simulink model "delayed_mpc_model"  (R2019a)
settings: Solver=FixedStepAuto  StartTime=0.0  StopTime=Tfinal  RelTol=1e-3
values from neighbouring files (symbols this model uses):
  A = [-0.0285 -0.0014; -0.0371 -0.1476]    [model.m]
  DCLINK_Cap = 1000e-12    (= 1e-09)    [mpc_model_parameters.m]    (also in mpc_model_parameters_dual_module.m = 0.001)
  FaultTime = 50    [mpc_model_parameters.m]
  FluxPM = MeanInducedVoltagePeak/(2*pi*100)    [mpc_model_parameters.m]    (also in mpc_model_parameters_dual_module.m)
  Inertia = 1e-2    (= 0.01)    [mpc_model_parameters.m]    (also in mpc_model_parameters_dual_module.m)
  iqrated = Trated/(1.5*PolePairs*FluxPM)    [mpc_model_parameters.m]    (also in mpc_model_parameters_dual_module.m)
  MeanLq = (1/12)*(Module1Phase_A_Lq+Module1Phase_B_Lq+Module1Phase_C_Lq+     Module2Phase_A_Lq+Module2Phase_B_Lq+Module2Phase_C_Lq+     Module3Phase_A_Lq+Module3Phase_B_Lq+Module3Phase_C_Lq+     Module4Phase_A_Lq+Module4Phase_B_Lq+Module4Phase_C_Lq)    [mpc_model_parameters.m]    (also in mpc_model_parameters_dual_module.m)
  PolePairs = 10    [mpc_model_parameters.m]    (also in mpc_model_parameters_dual_module.m)
  Rin = 1e-3    (= 0.001)    [mpc_model_parameters.m]    (also in mpc_model_parameters_dual_module.m)
  Rs = 0.531    [Loss_Distribution.m]    (also in MPC_id_iq.m; mpc_model_parameters.m = 0.321; mpc_model_parameters_dual_module.m = 0.539)
  Sampling_time = 1e-6    (= 1e-06)    [mpc_model_parameters.m]    (also in mpc_model_parameters_dual_module.m)
  SpeedRef1 = 50    [mpc_model_parameters.m]    (also in mpc_model_parameters_dual_module.m = 35)
  SpeedRef2 = 100    [mpc_model_parameters.m]    (also in mpc_model_parameters_dual_module.m = 35)
  SpeedRefUpdateTime = 0.25    [mpc_model_parameters.m]    (also in mpc_model_parameters_dual_module.m = 1.75)
  Tload1 = 5    [mpc_model_parameters.m]    (also in mpc_model_parameters_dual_module.m = 30)
  Tload2 = 10    [mpc_model_parameters.m]    (also in mpc_model_parameters_dual_module.m = 63.6619772368)
  TloadUpdateTime = 0.5    [mpc_model_parameters.m]    (also in mpc_model_parameters_dual_module.m)
  Vdc = 50    [mpc_model_parameters.m]    (also in mpc_model_parameters_dual_module.m = 40)
  Vin = Vdc + Rin*(Pout/Vdc)    (= 50.04)    [mpc_model_parameters.m]    (also in mpc_model_parameters_dual_module.m = 40.05)
  ViscousFriction = 1e-3    (= 0.001)    [mpc_model_parameters.m]    (also in mpc_model_parameters_dual_module.m)
undefined symbols (not defined in the file or in its folder): DiscIntNeverNeededParam
libraries: powerlib x16, dspswit3 x7, dspsigops x4, simulink x3, powerlib_meascontrol x2
settings Model: Creator=hakan  LastModifiedBy=hakan
settings SolverCC: ZeroCrossAlgorithm=Adaptive
settings DebuggingCC: IgnoredZcDiagnostic=none

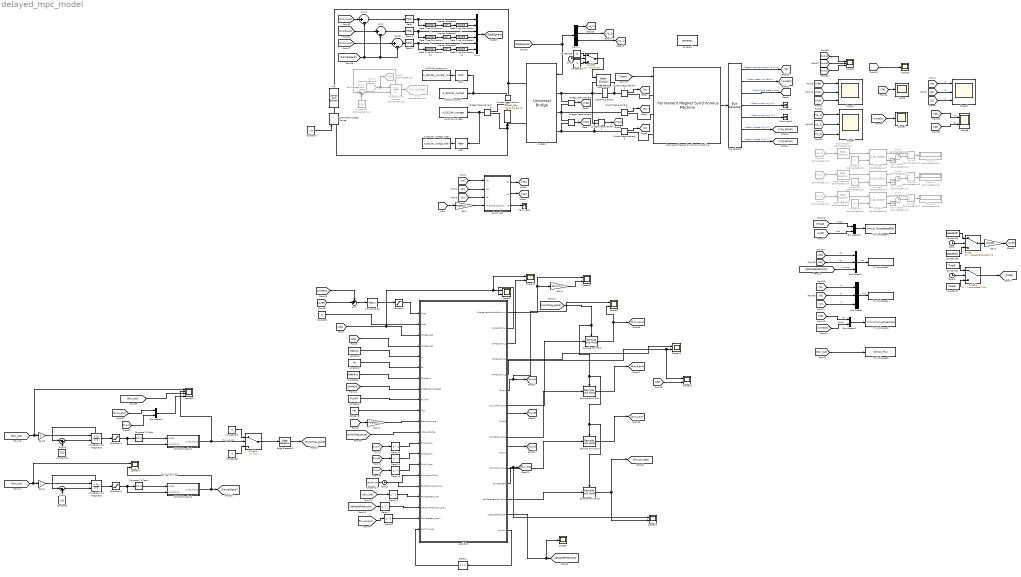
== system delayed_mpc_model ==
  A_DCLINK_current : ToWorkspace  VariableName=A_DCLINK_current  SaveFormat=Structure With Time  SampleTime=-1
  A_DCLINK_current_rms : ToWorkspace  VariableName=A_DCLINK_current_rms  SaveFormat=Structure With Time  SampleTime=-1
  A_DCLINK_voltage : ToWorkspace  VariableName=A_DCLINK_voltage  SaveFormat=Structure With Time  SampleTime=-1
  A_DCLINK_voltage_mean : ToWorkspace  VariableName=A_DCLINK_voltage_mean  SaveFormat=Structure With Time  SampleTime=-1
  Bus Creator : BusCreator  Inputs=3
  Bus Creator1 : BusCreator  Inputs=3
  Bus Creator2 : BusCreator  Inputs=2
  Bus Creator3 : BusCreator  Inputs=2
  Bus Creator4 : BusCreator  Inputs=2
  Bus Selector : BusSelector  OutputSignals=Electromagnetic torque Te (N*m),Rotor speed wm (rad/s),Rotor angle thetam (rad),Stator current is_q (A),Stator current is_d (A),Stator voltage Vs_q (V),Stator voltage Vs_d (V)
  Clock{,1..3} (4 alike) : Clock
  Clock4 : Clock  Commented=on
  Clock5 : Clock  Commented=on
  Clock6 : Clock  Commented=on
  Compare To Zero : simulink/Logic and Bit Operations/Compare To Zero  relop===  OutDataTypeStr=boolean
  Compare To Zero1 : simulink/Logic and Bit Operations/Compare To Zero  relop===  OutDataTypeStr=boolean
  Constant : Constant  Value=Vin
  Constant1 : Constant  Value=0
  Constant10 : Constant  Value=SpeedRef1
  Constant11 : Constant  Value=SpeedRef2
  Constant12 : Constant  Value=Tload2
  Constant15 : Constant  Value=0
  Constant16 : Constant
  Constant17 : Constant  Value=FaultTime
  Constant18 : Constant  Commented=on  Value=0
  Constant19 : Constant  Commented=on  Value=0
  Constant2 : Constant  Value=MeanLq
  Constant20 : Constant  Commented=on  Value=0
  Constant24 : Constant  Value=1.02
  Constant26 : Constant  Commented=on  Value=1.04
  Constant29 : Constant  Value=0
  Constant3 : Constant  Value=1.02
  Constant30 : Constant
  Constant5 : Constant  Value=Rs
  Constant6 : Constant  Value=PolePairs
  Constant7 : Constant  Value=FluxPM
  Constant8 : Constant  Value=Tload1
  Constant9 : Constant  Value=Vdc
  Controlled Voltage Source : powerlib/Electrical Sources/Controlled Voltage Source  Initialize=on  Source_Type=DC  Amplitude=Vin  Phase=0  Frequency=0  Measurements=None
      settings: SourceProductName=Simscape Electrical
  Counter : dspswit3/Counter  Commented=on  Direction=Up  CountEvent=Rising edge  CounterSize=User defined  MaxCount=9999999999999999999  InitialCount=0  Output=Count and Hit  HitValue=32  ResetInput=on  SamplesPerFrame=1  Ts=1  CntDtype=double  HitDtype=Logical
  Counter1 : dspswit3/Counter  Commented=on  Direction=Up  CountEvent=Rising edge  CounterSize=User defined  MaxCount=9999999999999999999  InitialCount=0  Output=Count and Hit  HitValue=32  ResetInput=on  SamplesPerFrame=1  Ts=1  CntDtype=double  HitDtype=Logical
  Counter2 : dspswit3/Counter  Commented=on  Direction=Up  CountEvent=Rising edge  CounterSize=User defined  MaxCount=9999999999999999999  InitialCount=0  Output=Count and Hit  HitValue=32  ResetInput=on  SamplesPerFrame=1  Ts=1  CntDtype=double  HitDtype=Logical
  Current Measurement{,1..3} (4 alike) : powerlib/Measurements/Current Measurement  PhasorSimulation=off  OutputType=Complex  PSBequivalent=0
      settings: SourceProductName=Simscape Electrical
  DCLINK_Cap : powerlib/Elements/Series RLC Branch  LConnTagsString=__new0  RConnTagsString=__new0  BranchType=C  Resistance=1  Inductance=1e-3  SetiL0=off  InitialCurrent=0  Capacitance=DCLINK_Cap  Setx0=on  InitialVoltage=Vin  Measurements=None
      settings: SourceProductName=Simscape Electrical
  Data Type Conversion10 : DataTypeConversion  OutDataTypeStr=boolean
  Data Type Conversion11 : DataTypeConversion  OutDataTypeStr=double
  Data Type Conversion6 : DataTypeConversion  OutDataTypeStr=boolean
  Data Type Conversion7 : DataTypeConversion  OutDataTypeStr=double
  Data Type Conversion8 : DataTypeConversion  OutDataTypeStr=boolean
  Data Type Conversion9 : DataTypeConversion  OutDataTypeStr=double
  Delay{1..2,5,11..14} (7 alike) : Delay  DelayLength=1
  Demux : Demux  Outputs=6
  Discrete-Time Integrator : DiscreteIntegrator  Commented=on  ExternalReset=falling  SampleTime=-1  ShowStatePort=on  ICPrevOutput=DiscIntNeverNeededParam  ICPrevScaledInput=DiscIntNeverNeededParam
  Discrete-Time Integrator1 : DiscreteIntegrator  ExternalReset=falling  SampleTime=Sampling_time  UpperSaturationLimit=1  LowerSaturationLimit=0  ShowStatePort=on  ICPrevOutput=DiscIntNeverNeededParam  ICPrevScaledInput=DiscIntNeverNeededParam
  Discrete-Time Integrator2 : DiscreteIntegrator  ExternalReset=falling  SampleTime=Sampling_time  UpperSaturationLimit=1  LowerSaturationLimit=0  ShowStatePort=on  ICPrevOutput=DiscIntNeverNeededParam  ICPrevScaledInput=DiscIntNeverNeededParam
  Display1 : Display  Commented=on
  Display2 : Display  Commented=on
  Display3 : Display  Commented=on
  Divide : Product  Commented=on  Inputs=*/
  Divide1 : Product  Commented=on  Inputs=*/
  Divide2 : Product  Commented=on  Inputs=*/
  Edge Detector : dspswit3/Edge Detector  Commented=on  InputProcessing=Columns as channels (frame based)
      settings: SourceProductName=DSP System Toolbox  SourceProductBaseCode=DS
  Edge Detector1 : dspswit3/Edge Detector  Commented=on  InputProcessing=Columns as channels (frame based)
      settings: SourceProductName=DSP System Toolbox  SourceProductBaseCode=DS
  Edge Detector2 : dspswit3/Edge Detector  Commented=on  InputProcessing=Columns as channels (frame based)
      settings: SourceProductName=DSP System Toolbox  SourceProductBaseCode=DS
  Edge Detector3 : dspswit3/Edge Detector  InputProcessing=Columns as channels (frame based)
      settings: SourceProductName=DSP System Toolbox  SourceProductBaseCode=DS
  From40 : From  Commented=on  GotoTag=va_1
  From41 : From  Commented=on  GotoTag=vb_1
  From42 : From  Commented=on  GotoTag=vc_1
  From72 : From  Commented=on  GotoTag=fsw_out
  Gain : Gain  Gain=PolePairs
  Gain1 : Gain  Gain=2*pi/60
  Gain2 : Gain  Gain=2
  Gain3 : Gain  Gain=PolePairs
  Gain4 : Gain  Gain=360/(2*pi)
  Gain8 : Gain  Gain=2
  Goto29 : Goto  Commented=on  GotoTag=fsw
  Goto9 : Goto  Commented=on  GotoTag=CarrierSignal
  Ideal Switch : powerlib/Power Electronics/Ideal Switch  Ron=0.001  Lon=0  IC=0  Rs=1e5  Cs=inf  Measurements=on
      settings: SourceProductName=Simscape Electrical
  Inverter1 : powerlib/Power Electronics/Universal Bridge  Arms=3  SnubberResistance=1e5  SnubberCapacitance=inf  Device=IGBT / Diodes  Ron=0.65e-3  Lon=0  ForwardVoltages="[  0  0  ]"  ForwardVoltage=0  GTOparameters=[ 10e-6 , 20e-6 ]  IGBTparameters=[ 1e-6 , 2e-6 ]  Measurements=All voltages and currents  Measurements_2=None  converterType=Rectifier
      settings: SourceProductName=Simscape Electrical
  Logical Operator3 : Logic  Operator=NOT  AllPortsSameDT=off  OutDataTypeStr=boolean
  Logical Operator4 : Logic  Operator=NOT  AllPortsSameDT=off  OutDataTypeStr=boolean
  Logical Operator5 : Logic  Operator=NOT  AllPortsSameDT=off  OutDataTypeStr=boolean
  MATLAB Function1 : MATLAB Function  TreatAsAtomicUnit=on
  MATLAB Function2 : MATLAB Function  TreatAsAtomicUnit=on
  Mean : powerlib_meascontrol/Measurements/Mean  Freq=THD_mean_frequency  Vinit=0  Ts=0
      settings: SourceProductName=Simscape Electrical
  Mux4 : Mux  Inputs=6
  PID Controller : simulink/Continuous/PID Controller  Controller=PID  Form=Parallel  TimeDomain=Continuous-time  SampleTime=-1  IntegratorMethod=Forward Euler  FilterMethod=Forward Euler  ControllerParametersSource=internal  P=1  I=10  D=0  UseFilter=on  N=100  TunerSelectOption=Transfer Function Based (PID Tuner App)  InitialConditionSource=internal  InitialConditionForIntegrator=0  InitialConditionForFilter=0  DifferentiatorICPrevScaledInput=0  ExternalReset=none  TrackingMode=off  Kt=1  LimitOutput=off  UpperSaturationLimit=inf  LowerSaturationLimit=-inf  LinearizeAsGain=on  AntiWindupMode=none  Kb=1  POutMin=[]  POutMax=[]  IOutMin=[]  IOutMax=[]  DOutMin=[]  DOutMax=[]  NOutMin=[]  NOutMax=[]  SumOutMin=[]  SumOutMax=[]  SaturationOutMin=[]  SaturationOutMax=[]  PParamMin=[]  PParamMax=[]  IParamMin=[]  IParamMax=[]  DParamMin=[]  DParamMax=[]  NParamMin=[]  NParamMax=[]  KbParamMin=[]  KbParamMax=[]  KtParamMin=[]  KtParamMax=[]  KbOutMin=[]  KbOutMax=[]  KtOutMin=[]  KtOutMax=[]  IntegratorOutMin=[]  IntegratorOutMax=[]  FilterOutMin=[]  FilterOutMax=[]  SumI1OutMin=[]  SumI1OutMax=[]  SumI2OutMin=[]  SumI2OutMax=[]  SumI3OutMin=[]  SumI3OutMax=[]  SumI4OutMin=[]  SumI4OutMax=[]  SumDOutMin=[]  SumDOutMax=[]  DifferentiatorOutMin=[]  DifferentiatorOutMax=[]  FilterDiffOutCoefMin=[]  FilterDiffOutCoefMax=[]  ReciprocalOutMin=[]  ReciprocalOutMax=[]  SumDenOutMin=[]  SumDenOutMax=[]  SumNumOutMin=[]  SumNumOutMax=[]  DivideOutMin=[]  DivideOutMax=[]  IntegratorContinuousStateAttributes=''  IntegratorStateMustResolveToSignalObject=off  IntegratorRTWStateStorageClass=Auto  FilterContinuousStateAttributes=''  FilterStateMustResolveToSignalObject=off  FilterRTWStateStorageClass=Auto  ParallelPVariant=InternalParameters  IdealPVariant=Disabled  IVariant=InternalParameters  DVariant=InternalParameters  IntegratorVariant=Continuous  SatVariant=Disabled  AWVariant=Passthrough  PCopyVariant=Disabled  TRVariant=Disabled  FdbkBlocksVariant=Forward  IdealPFdbkVariant=Disabled  SatFdbkVariant=Disabled  DerivativeFilterVariant=ContFilter  NVariant=InternalParameters  NCopyVariant=Disabled  FilterICVariant=InternalICsFilter  IntegratorICVariant=InternalICs  ExternalResetVariant=Disabled  TRSumVariant=Passthrough  SumFdbkVariant=Disabled  SumVariant=Sum_PID
  Permanent Magnet Synchronous Machine : powerlib/Machines/Permanent Magnet Synchronous Machine  NbPhases=3  FluxDistribution=Sinusoidal  RotorType=Round  MechanicalLoad=Torque Tm  PresetModel=No  ShowDetailedParameters=on  MeasurementBus=off  Resistance=Rs  Inductance=8.5e-3  dqInductances=[3.1e-3,3.6e-3]  La=Ls  MachineConstant=Voltage Constant (V_peak L-L / krpm)  Flux=0.18074  VoltageCst=VoltageConstant  TorqueCst=2.7111  Flat=120  Mechanical=[Inertia ViscousFriction PolePairs 0]  PolePairs=4  InitialConditions=[0*100*2*pi/60,0, 0,0]  InitialConditions5ph=[0 0 0 0 0 0]  TsPowergui=0  TsBlock=-1  RefAngle=90 degrees behind phase A axis (modified Park)
  RMS1 : powerlib_meascontrol/Measurements/RMS  TrueRMS=on  Freq=Load_Nominal_Freq  RMSInit=10  Ts=0
      settings: SourceProductName=Simscape Electrical
  Relay : Relay
  Relay1 : Relay
  Relay2 : Relay
  Rin : powerlib/Elements/Series RLC Branch  LConnTagsString=__new0  RConnTagsString=__new0  BranchType=R  Resistance=Rin  Inductance=1e-3  SetiL0=off  InitialCurrent=0  Capacitance=1000e-6  Setx0=off  InitialVoltage=0  Measurements=None
      settings: SourceProductName=Simscape Electrical
  Sample and Hold{,1..3} (4 alike) : dspsigops/Sample and Hold  trig=Rising edge  initCond=0  latchinput=off
  Saturation : Saturate  UpperLimit=2*iqrated  LowerLimit=-2*iqrated  LinearizeAsGain=off
  Saturation1 : Saturate  UpperLimit=1  LowerLimit=0
  Saturation2 : Saturate  UpperLimit=1  LowerLimit=0
  Scope{,1,5..6} (4 alike) : Scope
  Scope{8..15,17} (9 alike) : Scope  NumInputPorts=2
  Scope16 : Scope  NumInputPorts=4
  Scope{2..4,7} (4 alike) : Scope  NumInputPorts=3
  Series RLC Branch : powerlib/Elements/Series RLC Branch  LConnTagsString=__new0  RConnTagsString=__new0  BranchType=R  Resistance=5000  Inductance=1e-3  SetiL0=off  InitialCurrent=0  Capacitance=1e-6  Setx0=off  InitialVoltage=0  Measurements=None
      settings: SourceProductName=Simscape Electrical
  Sum : Sum  Inputs=-+|
  Sum1 : Sum  Inputs=|+-
  Sum10 : Sum  Inputs=|-+
  Sum2 : Sum  Inputs=|+-
  Sum3 : Sum  Commented=on  Inputs=|-+
  Sum4 : Sum  Inputs=|-+
  Sum5 : Sum  Inputs=|+-
  Switch : Switch  Criteria=u2 > Threshold  Threshold=SpeedRefUpdateTime
  Switch1 : Switch  Criteria=u2 > Threshold  Threshold=TloadUpdateTime
  Switch3 : Switch  Criteria=u2 > Threshold  Threshold=FaultTime
  Switch4 : Switch  Criteria=u2 ~= 0
  Terminator : Terminator
  Terminator1 : Terminator  Commented=on
  Terminator2 : Terminator  Commented=on
  Terminator3 : Terminator  Commented=on
  Terminator4 : Terminator
  Terminator5 : Terminator
  To Workspace1 : ToWorkspace  VariableName=Simout_PhaseCurrents_abc  SaveFormat=Timeseries  SampleTime=-1
  To Workspace2 : ToWorkspace  VariableName=Simout_PhaseCurrents_dq  SaveFormat=Timeseries  SampleTime=-1
  To Workspace3 : ToWorkspace  VariableName=Simout_TorqueSpeedMeas  SaveFormat=Timeseries  SampleTime=-1
  To Workspace4 : ToWorkspace  VariableName=Simout_TorqueSpeedRef  SaveFormat=Timeseries  SampleTime=-1
  To Workspace5 : ToWorkspace  VariableName=Simout_Fsw  SaveFormat=Timeseries  SampleTime=-1
  Voltage Measurement{,1..3} (4 alike) : powerlib/Measurements/Voltage Measurement  PhasorSimulation=off  OutputType=Complex  PSBequivalent=0
      settings: SourceProductName=Simscape Electrical
  abc to dq0 : MATLAB Function  TreatAsAtomicUnit=on
  powergui : powerlib/powergui  Priority=1  SimulationMode=Discrete  SampleTime=Sampling_time  frequency=60  Iterations=50  frequencyindice=0  Pbase=100e6  ErrMax=1e-4  UnitsV=kV  UnitsW=MW  buscounter=0  FunctionMessages=off  echomessages=off  EnableUseOfTLC=off  CurrentSourceSwitches=off  DisableSnubberDevices=off  DisableRonSwitches=off  DisableVfSwitches=off  DisplayEquations=off  AutomaticDiscreteSolvers=off  SolverType=Tustin/Backward Euler (TBE)  Interpol=off  ExternalGateDelay=off  methode=off  Ts=100  x0status=blocks  SPID=on  SwTol=0  HookPort=off  NonlinearTolerance=0  nMaxIteration=15  ContinueOnMaxIteration=off  RestoreLinks=warning  ResistiveCurrentMeasurement=off  Frange=[0:2:500]  Ylog=off  Xlog=on  ShowGrid=off  save=off  variable=ZData  structure=0  ZoomFFT=off  StartTime=0.0  cycles=1  DisplayStyle=1  fundamental=60  FreqAxis=off  MaxFrequency=1000  frequencyindicesteady=1  RmsSteady=1  display=off
      settings: SourceProductName=Simscape Electrical
  prediction : MATLAB Function  TreatAsAtomicUnit=on
  wires:
  Voltage Measurement3/1 -> Mean/1, A_DCLINK_voltage/1
  RMS1/1 -> A_DCLINK_current_rms/1
  Constant/1 -> Controlled Voltage Source/1
  Mean/1 -> A_DCLINK_voltage_mean/1
  Current Measurement/1 -> RMS1/1, A_DCLINK_current/1
  Permanent Magnet Synchronous Machine/1 -> Bus Selector/1
  Bus Selector/1 -> [Te]  "<Electromagnetic torque Te (N*m)>"
  Bus Selector/2 -> [wmech]  "<Rotor speed wm (rad/s)>"
  Current Measurement1/1 -> [Ia]
  Current Measurement2/1 -> [Ib]
  Current Measurement3/1 -> [Ic]
  Bus Selector/3 -> [thetam]  "<Rotor angle thetam (rad)>"
  [thetam] -> Gain/1
  [Ia] -> abc to dq0/1(ias)
  [Ib] -> abc to dq0/2(ibs)
  [Ic] -> abc to dq0/3(ics)
  Gain/1 -> abc to dq0/4(ref_frame_position)
  Bus Selector/4 -> Terminator4/1  "<Stator current is_q (A)>"
  Bus Selector/5 -> Terminator5/1  "<Stator current is_d (A)>"
  abc to dq0/2(iqs) -> [iqs]
  abc to dq0/1(ids) -> [ids]
  abc to dq0/3(i0) -> Terminator/1
  Constant2/1 -> prediction/5(Ls)
  Voltage Measurement/1 -> [Vab]
  Voltage Measurement1/1 -> [Vbc]
  Voltage Measurement2/1 -> [Vca]
  Bus Selector/6 -> [vsq_actual]  "<Stator voltage Vs_q (V)>"
  Bus Selector/7 -> [vsd_actual]  "<Stator voltage Vs_d (V)>"
  [Vca] -> Scope2/3
  [Vbc] -> Scope2/2
  [Vab] -> Scope2/1
  Constant5/1 -> prediction/6(Rs)
  Constant6/1 -> prediction/7(PolePairs)
  [wmech] -> prediction/8(ShaftAngularSpeed)
  Constant7/1 -> prediction/9(FluxPM)
  Constant9/1 -> prediction/10(Vdc)
  Gain3/1 -> prediction/11(ElectricalAngle)
  [thetam] -> Gain3/1
  [Tload] -> Permanent Magnet Synchronous Machine/1
  PID Controller/1 -> Saturation/1
  Sum/1 -> PID Controller/1
  [wmech] -> Sum/1
  [iqs] -> Bus Creator1/2  "iqs"
  [ids] -> Bus Creator1/1  "ids"
  Constant10/1 -> Switch/3
  Constant11/1 -> Switch/1
  Switch/1 -> Gain1/1
  Clock/1 -> Switch/2
  Clock1/1 -> Switch1/2
  Constant12/1 -> Switch1/1
  Constant8/1 -> Switch1/3
  Switch1/1 -> [Tload]
  Bus Creator/1 -> To Workspace1/1  "Iabc"
  Bus Creator1/1 -> To Workspace2/1  "Idq"
  Bus Creator2/1 -> To Workspace3/1
  [wref] -> Sum/2
  Gain1/1 -> [wref]
  [Tload] -> Bus Creator3/1  "Tload"
  [wref] -> Bus Creator3/2  "wref"
  Bus Creator3/1 -> To Workspace4/1
  [switching_pulse] -> prediction/12(InterruptPulse)
  Clock2/1 -> Switch3/2
  Constant15/1 -> Switch3/1
  Constant16/1 -> Switch3/3
  Switch3/1 -> Ideal Switch/1
  Clock3/1 -> prediction/16(SimulationClock)
  Constant17/1 -> prediction/17(FaultOccuranceTime)
  [va_1] -> Scope7/1
  [vb_1] -> Scope7/2
  [vc_1] -> Scope7/3
  Edge Detector/1 -> Counter/1
  Constant18/1 -> Counter/2
  Counter/1 -> Divide/1
  Clock4/1 -> Divide/2
  Divide/1 -> Display2/1
  [Ib] -> Bus Creator/2  "Ib"
  [Ia] -> Bus Creator/1  "Ia"
  [Ic] -> Bus Creator/3  "Ic"
  [Ib] -> Scope3/2  "Ib"
  [Ic] -> Scope3/3  "Ic"
  [Ia] -> Scope3/1  "Ia"
  [iqs] -> Scope8/1  "iqs"
  [ids] -> Scope8/2  "ids"
  Counter/2 -> Terminator1/1
  From40/1 -> Edge Detector/1
  From41/1 -> Edge Detector1/1
  Counter1/2 -> Terminator2/1
  Divide1/1 -> Display1/1
  Clock5/1 -> Divide1/2
  Counter1/1 -> Divide1/1
  Constant19/1 -> Counter1/2
  Edge Detector1/1 -> Counter1/1
  Edge Detector2/1 -> Counter2/1
  Constant20/1 -> Counter2/2
  Counter2/1 -> Divide2/1
  Clock6/1 -> Divide2/2
  Divide2/1 -> Display3/1
  Counter2/2 -> Terminator3/1
  From42/1 -> Edge Detector2/1
  [Te] -> Bus Creator2/1  "Te"
  [wmech] -> Bus Creator2/2  "wmech"
  [Te] -> Scope/1
  [wmech] -> Scope1/1
  [DutyB] -> Scope4/2
  [DutyA] -> Scope4/1
  [DutyC] -> Scope4/3
  Constant26/1 -> Sum3/2
  From72/1 -> Goto29/1, Discrete-Time Integrator/1
  Discrete-Time Integrator/State -> Sum3/1
  Sum3/1 -> Discrete-Time Integrator/2
  [GateSignals] -> Inverter1/1, Demux/1
  Demux/1 -> [va_1]
  Demux/3 -> [vb_1]
  Delay11/1 -> prediction/18(FswSelected_prev)
  [fsw_out] -> Delay11/1
  [DutyB] -> Delay13/1
  [DutyA] -> Delay12/1
  [DutyC] -> Delay14/1
  Delay13/1 -> prediction/14(DutyB_prev)
  Delay12/1 -> prediction/13(DutyA_prev)
  Delay14/1 -> prediction/15(DutyC_prev)
  Discrete-Time Integrator/1 -> Goto9/1
  Demux/5 -> [vc_1]
  prediction/14(IqRipplePrediction) -> Scope6/1, [IqRipplePrediction]
  [IqRipplePrediction] -> Delay1/1
  Delay1/1 -> prediction/19(IqRipplePrediction_prev)
  [CarrierSignal] -> Sum1/2, Sum2/2, Sum5/2
  Logical Operator4/1 -> Data Type Conversion9/1
  [DutyA_app] -> Sum1/1
  Data Type Conversion8/1 -> Logical Operator4/1
  Data Type Conversion10/1 -> Logical Operator5/1
  Relay1/1 -> Data Type Conversion8/1, Mux4/3
  Relay2/1 -> Data Type Conversion10/1, Mux4/5
  Data Type Conversion6/1 -> Logical Operator3/1
  Sum1/1 -> Relay/1
  Data Type Conversion11/1 -> Mux4/6
  [DutyC_app] -> Sum5/1
  Relay/1 -> Mux4/1, Data Type Conversion6/1
  Data Type Conversion9/1 -> Mux4/4
  Sum5/1 -> Relay2/1
  Logical Operator3/1 -> Data Type Conversion7/1
  Logical Operator5/1 -> Data Type Conversion11/1
  Sum2/1 -> Relay1/1
  Mux4/1 -> [GateSignals]
  [DutyB_app] -> Sum2/1
  Data Type Conversion7/1 -> Mux4/2
  [fsw_out] -> Scope5/1
  Saturation/1 -> prediction/1(iqref)
  Discrete-Time Integrator2/State -> Sum10/1
  Gain8/1 -> Discrete-Time Integrator2/1
  Sum10/1 -> Discrete-Time Integrator2/2
  [fsw_out] -> Scope16/1, Gain8/1
  Saturation1/1 -> MATLAB Function1/2(inputwave), Compare To Zero/1
  Constant24/1 -> Sum10/2
  Discrete-Time Integrator2/1 -> Saturation1/1
  Compare To Zero/1 -> MATLAB Function1/1(pulse)
  [fsw_out] -> To Workspace5/1
  [IqRipplePrediction] -> Bus Creator1/3  "iqripple"
  Delay5/1 -> prediction/20(FswSelected_prev1)
  [fsw_out_app] -> Delay5/1
  [switching_pulse] -> Sample and Hold3/Trigger, Sample and Hold2/Trigger, Sample and Hold1/Trigger, Sample and Hold/Trigger
  Sample and Hold/1 -> Scope11/2, [DutyA_app]
  Sample and Hold1/1 -> [DutyB_app]
  Sample and Hold2/1 -> [DutyC_app]
  Sample and Hold3/1 -> Scope10/2, [fsw_out_app]
  prediction/7(DutyAPrevValue) -> Sample and Hold/1
  prediction/9(DutyBPrevValue) -> Sample and Hold1/1
  prediction/11(DutyCPrevValue) -> Sample and Hold2/1
  prediction/13(FswSelectedPrevValue) -> Sample and Hold3/1
  prediction/6(DutyA) -> [DutyA], Scope11/1
  prediction/8(DutyB) -> [DutyB]
  prediction/10(DutyC) -> [DutyC]
  prediction/12(FswSelected) -> Scope10/1, [fsw_out]
  Constant1/1 -> prediction/2(idref)
  prediction/2(IqPrediction_1) -> Scope9/2
  prediction/3(IqPrediction_2) -> Scope12/2
  Switch4/1 -> Edge Detector3/1
  MATLAB Function1/1(outputwave) -> Scope16/2, Switch4/2  "fsw_out_car"
  Constant30/1 -> Switch4/3
  Constant29/1 -> Switch4/1
  Compare To Zero1/1 -> MATLAB Function2/1(pulse)
  Discrete-Time Integrator1/1 -> Saturation2/1
  Constant3/1 -> Sum4/2
  Saturation2/1 -> Compare To Zero1/1, MATLAB Function2/2(inputwave)
  [fsw_out] -> Scope14/1, Gain2/1
  Sum4/1 -> Discrete-Time Integrator1/2
  Gain2/1 -> Discrete-Time Integrator1/1
  Discrete-Time Integrator1/State -> Sum4/1
  MATLAB Function2/1(outputwave) -> Scope14/2, [CarrierSignal]  "fsw_out_app_car"
  [ids] -> Scope12/1, Scope9/1, prediction/3(IdMeasured)
  [iqs] -> prediction/4(IqMeasured)
  prediction/15(dummy) -> Delay2/1
  Delay2/1 -> prediction/21(dummy_prev)
  Edge Detector3/1 -> [switching_pulse]
  prediction/4(IdPrediction_1) -> Scope13/1
  prediction/5(IdPrediction_2) -> Scope15/1, Scope13/2
  [ids] -> Scope15/2
  [fsw_out] -> Scope16/3
  [DutyA_app] -> Bus Creator4/1
  [DutyA] -> Bus Creator4/2
  Bus Creator4/1 -> Scope16/4
  prediction/1(VoltageVectorAngleOptimum) -> Gain4/1, Scope17/1
  Gain4/1 -> Scope17/2
  connections:
  Rin/LConn1 -- Current Measurement/RConn1 -- Inverter1/RConn1
  Controlled Voltage Source/LConn1 -- Voltage Measurement3/LConn2 -- DCLINK_Cap/RConn1 -- Inverter1/RConn2
  DCLINK_Cap/LConn1 -- Current Measurement/LConn1 -- Voltage Measurement3/LConn1
  Controlled Voltage Source/RConn1 -- Rin/RConn1
  Voltage Measurement2/LConn2 -- Ideal Switch/LConn1 -- Series RLC Branch/LConn1 -- Voltage Measurement/LConn1 -- Inverter1/LConn1
  Current Measurement2/LConn1 -- Voltage Measurement1/LConn1 -- Voltage Measurement/LConn2 -- Inverter1/LConn2
  Inverter1/LConn3 -- Voltage Measurement1/LConn2 -- Voltage Measurement2/LConn1 -- Current Measurement3/LConn1
  Current Measurement3/RConn1 -- Permanent Magnet Synchronous Machine/LConn3
  Permanent Magnet Synchronous Machine/LConn2 -- Current Measurement2/RConn1
  Permanent Magnet Synchronous Machine/LConn1 -- Current Measurement1/RConn1
  Current Measurement1/LConn1 -- Ideal Switch/RConn1 -- Series RLC Branch/RConn1

== matlab function delayed_mpc_model/prediction ==
  data: VoltageVectorAngleOptimum output; IqPrediction_1 output; IqPrediction_2 output; IdPrediction_1 output; IdPrediction_2 output; DutyA output; DutyAPrevValue output; DutyB output; DutyBPrevValue output; DutyC output; DutyCPrevValue output; iqref input; idref input; IdMeasured input; IqMeasured input; Ls input; Rs input; PolePairs input; ShaftAngularSpeed input; FluxPM input; Vdc input; ElectricalAngle input; InterruptPulse input; DutyA_prev input; DutyB_prev input; DutyC_prev input; SimulationClock input; FaultOccuranceTime input; FswSelected_prev input; FswSelected output; FswSelectedPrevValue output; IqRipplePrediction output; IqRipplePrediction_prev input; FswSelected_prev1 input; dummy_prev input; dummy output
function [VoltageVectorAngleOptimum,IqPrediction_1,IqPrediction_2,IdPrediction_1,IdPrediction_2,DutyA,DutyAPrevValue, DutyB,DutyBPrevValue, DutyC,DutyCPrevValue, FswSelected,FswSelectedPrevValue, IqRipplePrediction,dummy]  = fcn(iqref,idref,IdMeasured, IqMeasured, Ls, Rs,PolePairs,ShaftAngularSpeed,FluxPM,Vdc,ElectricalAngle,InterruptPulse,DutyA_prev, DutyB_prev, DutyC_prev, SimulationClock,FaultOccuranceTime,FswSelected_prev, IqRipplePrediction_prev,FswSelected_prev1,dummy_prev)
Ld = Ls;
Lq = Ls;
I_Normalize = 11.7362; %this is the rated value of the IqMeasured
cost = zeros(1,8);
VdPrediction_1 = zeros(1,8);
VqPrediction_1 = zeros(1,8);
% FswOptions = [5000; 10000; 15000; 20000; 25000; 30000; 35000; 40000];
FswMax = 40000;
FswOptions = 1000:1000:FswMax;
cost = zeros(1,numel(FswOptions));
VdPrediction_1 = zeros(1,numel(FswOptions));
VqPrediction_1 = zeros(1,numel(FswOptions));
VdPrediction_2 = zeros(1,numel(FswOptions));
VqPrediction_2 = zeros(1,numel(FswOptions));
IqRipplePredictionArray_1 = zeros(1,numel(FswOptions));
IqRipplePredictionArray_2 = zeros(1,numel(FswOptions));
VoltageDuring_T1_1 = zeros(1,numel(FswOptions));
VoltageDuring_T2_1 = zeros(1,numel(FswOptions));
VoltageDuring_T0_1 = zeros(1,numel(FswOptions));
VoltageDuring_T1_2 = zeros(1,numel(FswOptions));
VoltageDuring_T2_2 = zeros(1,numel(FswOptions));
VoltageDuring_T0_2 = zeros(1,numel(FswOptions));
MagnitudePrediction_1 = zeros(1,numel(FswOptions));
MagnitudePrediction_2 = zeros(1,numel(FswOptions));

SvpwmT1Prediction_1 =  zeros(1,numel(FswOptions));
SvpwmT2Prediction_1 =  zeros(1,numel(FswOptions));
SvpwmT0Prediction_1 =  zeros(1,numel(FswOptions));

SvpwmT1Prediction_2 =  zeros(1,numel(FswOptions));
SvpwmT2Prediction_2 =  zeros(1,numel(FswOptions));
SvpwmT0Prediction_2 =  zeros(1,numel(FswOptions));

ValfaPrediction_1 = zeros(1,numel(FswOptions)); 
VbetaPrediction_1 = zeros(1,numel(FswOptions)); 
maPrediction_1 = zeros(1,numel(FswOptions)); 

ValfaPrediction_2 = zeros(1,numel(FswOptions)); 
VbetaPrediction_2 = zeros(1,numel(FswOptions)); 
maPrediction_2 = zeros(1,numel(FswOptions)); 

IqDelta_Prediction_During_T1_1 =  zeros(1,numel(FswOptions));
IqDelta_Prediction_During_T2_1 =  zeros(1,numel(FswOptions));
IqDelta_Prediction_During_T0_1 =  zeros(1,numel(FswOptions));
IqDelta_Prediction_During_T1_2 =  zeros(1,numel(FswOptions));
IqDelta_Prediction_During_T2_2 =  zeros(1,numel(FswOptions));
IqDelta_Prediction_During_T0_2 =  zeros(1,numel(FswOptions));
VoltageVectorAnglePredictionMod_1 = zeros(1,numel(FswOptions));
VoltageVectorAnglePrediction_1 = zeros(1,numel(FswOptions));
VoltageVectorAnglePredictionMod_2 = zeros(1,numel(FswOptions));
VoltageVectorAnglePrediction_2 = zeros(1,numel(FswOptions));

% DutyAToBeApplied = DutyAToBeApplied_prev;
% DutyBToBeApplied = DutyBToBeApplied_prev;
% DutyCToBeApplied = DutyCToBeApplied_prev;
IdPrediction_1 = 0;
IdPrediction_2 = 0;
IqPrediction_1 = 0;
IqPrediction_2 = 0;


IqRippleCoeff = 10000;
IqRefCoeff = 10000;
IdRefCoeff = 15;
FswCoeff = 1500;
DutyAPrevValue =0;
DutyBPrevValue =0;
DutyCPrevValue =0;
FswSelectedPrevValue = 0;
VoltageVectorAngleOptimum = 0;
% dummy = 0;
% A = [(1-Rs/(FswOptions(i)*Ls)) ShaftAngularSpeed/FswOptions(i); -ShaftAngularSpeed/FswOptions(i) (1-Rs/(FswOptions(i)*Ls))];
% B = [1/((FswOptions(i)*Ls)) 0 ; 1/((FswOptions(i)*Ls)) 0];
% E = [0 -FluxPm*ShaftAngularSpeed/(((FswOptions(i)*Ls)))];
        TheAngle = 0;
        angleoffset = 10*pi;
if(InterruptPulse==1)
   
    DutyAPrevValue = DutyA_prev;
    DutyBPrevValue = DutyB_prev;
    DutyCPrevValue = DutyC_prev;
    FswSelectedPrevValue = FswSelected_prev;
    for i = 1:numel(FswOptions)
        % calculate vd vq
        VdPrediction_1(i) = Rs*IdMeasured + Ld*FswOptions(i)*(idref-IdMeasured)-PolePairs*ShaftAngularSpeed*Lq*IqMeasured;
        VqPrediction_1(i) = Rs*IqMeasured + Lq*FswOptions(i)*(iqref-IqMeasured)+PolePairs*ShaftAngularSpeed*(Ld*IdMeasured+FluxPM);
        
        MagnitudePrediction_1(i) = sqrt(VdPrediction_1(i)^2+VqPrediction_1(i)^2);
        
%         TheAngle = PolePairs*ShaftAngularSpeed/FswOptions(i);

        ValfaPrediction_1(i) = sin(ElectricalAngle+TheAngle)*VdPrediction_1(i)+cos(ElectricalAngle+TheAngle)*VqPrediction_1(i);
        VbetaPrediction_1(i) =-cos(ElectricalAngle+TheAngle)*VdPrediction_1(i)+sin(ElectricalAngle+TheAngle)*VqPrediction_1(i);     
        
        VoltageVectorAnglePrediction_1(i) = atan2(VbetaPrediction_1(i),ValfaPrediction_1(i))+angleoffset;
        VoltageVectorAnglePredictionMod_1(i) = mod(VoltageVectorAnglePrediction_1(i),pi/3);
        
        maPrediction_1(i) = MagnitudePrediction_1(i)/(Vdc/sqrt(3));
        
        SvpwmT1Prediction_1(i) = (1/FswOptions(i))*maPrediction_1(i)*sin(pi/3-VoltageVectorAnglePredictionMod_1(i));
        SvpwmT2Prediction_1(i) = (1/FswOptions(i))*maPrediction_1(i)*sin(VoltageVectorAnglePredictionMod_1(i));
        SvpwmT0Prediction_1(i) = (1/FswOptions(i))-SvpwmT1Prediction_1(i)-SvpwmT2Prediction_1(i);        
        
        VoltageDuring_T1_1(i) = 2/3*Vdc-MagnitudePrediction_1(i);
        VoltageDuring_T2_1(i) = 2/3*Vdc-MagnitudePrediction_1(i);
        VoltageDuring_T0_1(i) = -MagnitudePrediction_1(i);
        
        IqDelta_Prediction_During_T1_1(i) = VoltageDuring_T1_1(i)*SvpwmT1Prediction_1(i)/Ls;
        IqDelta_Prediction_During_T2_1(i) = VoltageDuring_T2_1(i)*SvpwmT2Prediction_1(i)/Ls;
        IqDelta_Prediction_During_T0_1(i) = -VoltageDuring_T0_1(i)*SvpwmT0Prediction_1(i)/Ls;
        
        IqRipplePredictionArray_1(i) = IqDelta_Prediction_During_T1_1(i)+IqDelta_Prediction_During_T2_1(i)+IqDelta_Prediction_During_T0_1(i);
        
        %predict the future output
        IdPrediction_1 = IdMeasured + (1/FswOptions(i))*(VdPrediction_1(i)/Ld-Rs/Ld*IdMeasured+Lq/Ld*PolePairs*ShaftAngularSpeed*IqMeasured);
        IqPrediction_1 = IqMeasured + (1/FswOptions(i))*(VqPrediction_1(i)*Lq-Rs/Lq*IqMeasured-Ld/Lq*PolePairs*ShaftAngularSpeed*IdMeasured-FluxPM*PolePairs*ShaftAngularSpeed/Lq);
        
%         Ts = (1/FswOptions(i));
%         IdPrediction_1 = IdMeasured + (1/FswOptions(i))*IdMeasured*(1-Rs*Ts/Ls)+IqMeasured*Ts*ShaftAngularSpeed*Ts*PolePairs+VdPrediction_1(i)*Ts*Ts/Ls;
%         IqPrediction_1 = IqMeasured + Ts*IdMeasured*(-Ts*ShaftAngularSpeed*PolePairs) + Ts*IqMeasured*(1-Rs*Ts/Ls) + VqPrediction_1(i)*Ts*Ts/Ls-FluxPM*Ts*Ts*ShaftAngularSpeed*PolePairs/Ls;

%         Ts = (1/FswOptions(i));
%         IdPrediction_1 = (1-Ts*Rs/Ls)*IdMeasured+Ts*ShaftAngularSpeed*PolePairs*IqMeasured+Ts/Ls*VdPrediction_1(i);
%         IqPrediction_1 = (1-Ts*Rs/Ls)*IqMeasured-Ts*ShaftAngularSpeed*PolePairs*IdMeasured+Ts/Ls*VqPrediction_1(i);

        TePrediction_1 = 1.5*PolePairs*(FluxPM*IqPrediction_1+0*(Ld-Lq)*IdPrediction_1*IqPrediction_1); % reluctance torque component is multiplied by 0, since it caused unreasonable torque values.
        
        %%%%%%%%%%%%%%%%%%%begin - second prediction
        VdPrediction_2(i) = Rs*IdPrediction_1 + Ld*FswOptions(i)*(idref-IdPrediction_1)-PolePairs*ShaftAngularSpeed*Lq*IqPrediction_1;
        VqPrediction_2(i) = Rs*IqPrediction_1 + Lq*FswOptions(i)*(iqref-IqPrediction_1)+PolePairs*ShaftAngularSpeed*(Ld*IdPrediction_1+FluxPM);        

        MagnitudePrediction_2(i) = sqrt(VdPrediction_2(i)^2+VqPrediction_2(i)^2);
        
%         TheAngle = TheAngle + PolePairs*ShaftAngularSpeed/FswOptions(i);
%         TheAngle = 0;
        
        ValfaPrediction_2(i) = sin(ElectricalAngle+TheAngle)*VdPrediction_2(i)+cos(ElectricalAngle+TheAngle)*VqPrediction_2(i);
        VbetaPrediction_2(i) =-cos(ElectricalAngle+TheAngle)*VdPrediction_2(i)+sin(ElectricalAngle+TheAngle)*VqPrediction_2(i); 

        VoltageVectorAnglePrediction_2(i) = atan2(VbetaPrediction_2(i),ValfaPrediction_2(i))+angleoffset;
        VoltageVectorAnglePredictionMod_2(i) = mod(VoltageVectorAnglePrediction_2(i),pi/3);
        
        maPrediction_2(i) = MagnitudePrediction_2(i)/(Vdc/sqrt(3));
        
        SvpwmT1Prediction_2(i) = (1/FswOptions(i))*maPrediction_2(i)*sin(pi/3-VoltageVectorAnglePredictionMod_2(i));
        SvpwmT2Prediction_2(i) = (1/FswOptions(i))*maPrediction_2(i)*sin(VoltageVectorAnglePredictionMod_2(i));
        SvpwmT0Prediction_2(i) = (1/FswOptions(i))-SvpwmT1Prediction_2(i)-SvpwmT2Prediction_2(i);      
        
        VoltageDuring_T1_2(i) = 2/3*Vdc-MagnitudePrediction_2(i);
        VoltageDuring_T2_2(i) = 2/3*Vdc-MagnitudePrediction_2(i);
        VoltageDuring_T0_2(i) = -MagnitudePrediction_2(i);
        
        IqDelta_Prediction_During_T1_2(i) = VoltageDuring_T1_2(i)*SvpwmT1Prediction_2(i)/Ls;
        IqDelta_Prediction_During_T2_2(i) = VoltageDuring_T2_2(i)*SvpwmT2Prediction_2(i)/Ls;
        IqDelta_Prediction_During_T0_2(i) = -VoltageDuring_T0_2(i)*SvpwmT0Prediction_2(i)/Ls;  
        
        IqRipplePredictionArray_2(i) = IqDelta_Prediction_During_T1_2(i)+IqDelta_Prediction_During_T2_2(i)+IqDelta_Prediction_During_T0_2(i);
        
%         IdPrediction_2 = IdPrediction_1 + (1/FswOptions(i))*(VdPrediction_2(i)/Ld-Rs/Ld*IdPrediction_1+Lq/Ld*PolePairs*ShaftAngularSpeed*IqPrediction_1);
%         IqPrediction_2 = IqPrediction_1 + (1/FswOptions(i))*(VqPrediction_2(i)*Lq-Rs/Lq*IqPrediction_1-Ld/Lq*PolePairs*ShaftAngularSpeed*IdPrediction_1-FluxPM*PolePairs*ShaftAngularSpeed/Lq);

        IdPrediction_2 = IdMeasured + (1/FswOptions(i))*(VdPrediction_2(i)/Ld-Rs/Ld*IdMeasured+Lq/Ld*PolePairs*ShaftAngularSpeed*IqMeasured);
        IqPrediction_2 = IqMeasured + (1/FswOptions(i))*(VqPrediction_2(i)*Lq-Rs/Lq*IqMeasured-Ld/Lq*PolePairs*ShaftAngularSpeed*IdMeasured-FluxPM*PolePairs*ShaftAngularSpeed/Lq);
        
%         IdPrediction_2 = IdPrediction_1 + (1/FswOptions(i))*(VdPrediction_1(i)/Ld-Rs/Ld*IdPrediction_1+Lq/Ld*PolePairs*ShaftAngularSpeed*IqPrediction_1);
%         IqPrediction_2 = IqPrediction_1 + (1/FswOptions(i))*(VqPrediction_1(i)*Lq-Rs/Lq*IqPrediction_1-Ld/Lq*PolePairs*ShaftAngularSpeed*IdPrediction_1-FluxPM*PolePairs*ShaftAngularSpeed/Lq);        

%         IdPrediction_2 = IdPrediction_1 + (1/FswOptions(i))*IdPrediction_1*(1-Rs*Ts/Ls)+IqPrediction_1*Ts*ShaftAngularSpeed*Ts*PolePairs+VdPrediction_2(i)*Ts*Ts/Ls;
%         IqPrediction_2 = IqPrediction_1 + Ts*IdPrediction_1*(-Ts*ShaftAngularSpeed*PolePairs) + Ts*IqPrediction_1*(1-Rs*Ts/Ls) + VqPrediction_2(i)*Ts*Ts/Ls-FluxPM*Ts*Ts*ShaftAngularSpeed*PolePairs/Ls;

%         IdPrediction_2 = (1-Ts*Rs/Ls)*IdPrediction_1+Ts*ShaftAngularSpeed*PolePairs*IqPrediction_1+Ts/Ls*VdPrediction_1(i);
%         IqPrediction_2 = (1-Ts*Rs/Ls)*IqPrediction_1-Ts*ShaftAngularSpeed*PolePairs*IdPrediction_1+Ts/Ls*VqPrediction_1(i);        
        
        TePrediction_2 = 1.5*PolePairs*(FluxPM*IqPrediction_2+0*(Ld-Lq)*IdPrediction_2*IqPrediction_2); % reluctance torque component is multiplied by 0, since it caused unreasonable torque values.
        
        %%%%%%%%%%%%%%%%%%%end - second prediction
        
        
        %calculate the cost
%         if(abs(IqPrediction_1)>30)||(abs(TePrediction_1)>50)
%             ProtectionConstant = inf;
%         else
            ProtectionConstant = 0;
%         end
%         cost(i) = (IqRipplePredictionArray(i)/I_Normalize)^2*IqRippleCoeff+IqRefCoeff*((iqref-IqPrediction_1)/I_Normalize)^2+((idref-IdPrediction_1)/I_Normalize)^2*IdRefCoeff+ProtectionConstant+FswOptions(i)/FswMax*FswCoeff;%+IqRipplePrediction_prev^2*100000000;
%         cost(i) = (IqRipplePredictionArray_1(i)/I_Normalize)^2*IqRippleCoeff+IqRefCoeff*((iqref-IqPrediction_1)/I_Normalize)^2+((idref-IdPrediction_1)/I_Normalize)^2*IdRefCoeff+ProtectionConstant+FswOptions(i)/FswMax*FswCoeff;%+IqRipplePrediction_prev^2*100000000;
        cost(i) = (IqRipplePredictionArray_2(i)/I_Normalize)^2*IqRippleCoeff+IqRefCoeff*((iqref-IqPrediction_2)/I_Normalize)^2+((idref-IdPrediction_2)/I_Normalize)^2*IdRefCoeff+ProtectionConstant+FswOptions(i)/FswMax*FswCoeff;%+IqRipplePrediction_prev^2*100000000;
        
    end
    
    [CostMinVal, MinimumCostIndex] = min(cost);
    
    DutyA = 0;
    DutyB = 0;
    DutyC = 0;
%     VdsOptimum_1 = VdPrediction_1(MinimumCostIndex);
%     VqsOptimum_1 = VqPrediction_1(MinimumCostIndex);
    FswSelected = FswOptions(MinimumCostIndex);
    
% if(dummy_prev == 0)
    dummy = dummy_prev+1;
    if(dummy==3)
        dummy = 0;
    end
    if(dummy == 2)
%         FswSelected = 30000;
    end
    if(dummy == 1)
%         FswSelected = 20000;
    end
    if(dummy == 0)
%         FswSelected = 10000;
    end    
% else
%     dummy = 0;
% end
    TswSelected = 1/FswSelected;

    
    Svpwm_T1 = SvpwmT1Prediction_2(MinimumCostIndex);
    Svpwm_T2 = SvpwmT2Prediction_2(MinimumCostIndex);
    Svpwm_T0 = SvpwmT0Prediction_2(MinimumCostIndex);
    VoltageVectorAngleOptimum = mod(VoltageVectorAnglePrediction_2(MinimumCostIndex),2*pi);
    
    IqRipplePrediction = IqRipplePredictionArray_2(MinimumCostIndex);
    
    if (mod(VoltageVectorAngleOptimum, 2*pi)<=pi/3)&&(mod(VoltageVectorAngleOptimum, 2*pi)>=0)  % sector 1
        DutyA = (Svpwm_T1+Svpwm_T2+Svpwm_T0/2)/TswSelected;
        DutyB = (Svpwm_T2+Svpwm_T0/2)/TswSelected;
        DutyC = (Svpwm_T0/2)/TswSelected;
%         sectornumber = 1;
        return;
    end
    if (mod(VoltageVectorAngleOptimum, 2*pi)<=2*pi/3)&&(mod(VoltageVectorAngleOptimum, 2*pi)>=pi/3)  % sector 2
        DutyA = (Svpwm_T1+Svpwm_T0/2)/TswSelected;
        DutyB = (Svpwm_T1+Svpwm_T2+Svpwm_T0/2)/TswSelected;
        DutyC = (Svpwm_T0/2)/TswSelected;
%         sectornumber = 2;
        return;
    end
    if (mod(VoltageVectorAngleOptimum, 2*pi)<=pi)&&(mod(VoltageVectorAngleOptimum, 2*pi)>=2*pi/3)  % sector 3
        if(mod(VoltageVectorAngleOptimum, pi)==0)
            DutyA = (Svpwm_T0/2)/TswSelected;
            DutyB = (Svpwm_T1+Svpwm_T0/2)/TswSelected;
            DutyC = (Svpwm_T1+Svpwm_T2+Svpwm_T0/2)/TswSelected;
        else
            DutyA = (Svpwm_T0/2)/TswSelected;
            DutyB = (Svpwm_T1+Svpwm_T2+Svpwm_T0/2)/TswSelected;
            DutyC = (Svpwm_T2+Svpwm_T0/2)/TswSelected;
        end
%         sectornumber = 3;
        return;
    end
    if (mod(VoltageVectorAngleOptimum, 2*pi)<=4*pi/3)&&(mod(VoltageVectorAngleOptimum, 2*pi)>=pi)  % sector 4
        DutyA = (Svpwm_T0/2)/TswSelected;
        DutyB = (Svpwm_T1+Svpwm_T0/2)/TswSelected;
        DutyC = (Svpwm_T1+Svpwm_T2+Svpwm_T0/2)/TswSelected;
%         sectornumber = 4;
        return;
    end
    if (mod(VoltageVectorAngleOptimum, 2*pi)<=5*pi/3)&&(mod(VoltageVectorAngleOptimum, 2*pi)>=4*pi/3)  % sector 5
        DutyA = (Svpwm_T2+Svpwm_T0/2)/TswSelected;
        DutyB = (Svpwm_T0/2)/TswSelected;
        DutyC = (Svpwm_T1+Svpwm_T2+Svpwm_T0/2)/TswSelected;
%         sectornumber = 5;
        return;
    end
    if (mod(VoltageVectorAngleOptimum, 2*pi)<=2*pi)&&(mod(VoltageVectorAngleOptimum, 2*pi)>=5*pi/3)  % sector 6
        DutyA = (Svpwm_T1+Svpwm_T2+Svpwm_T0/2)/TswSelected;
        DutyB = (Svpwm_T0/2)/TswSelected;
        DutyC = (Svpwm_T1+Svpwm_T0/2)/TswSelected;
%         sectornumber = 6;
        return;
    end

else %switching pulse
    
    FswSelected = FswSelected_prev;
    DutyA = DutyA_prev;
    DutyB = DutyB_prev;
    DutyC = DutyC_prev;
    IqRipplePrediction = IqRipplePrediction_prev;
    dummy = dummy_prev;

end

== matlab function delayed_mpc_model/MATLAB Function2 ==
  data: pulse input; inputwave input; outputwave output
function outputwave  = fcn(pulse, inputwave)

persistent state

if isempty(state)
state = 0;
end

if(pulse==1)
    state = state +1;
end

if(mod(state,2)==1)
    outputwave = inputwave;
    return;
end
if(mod(state,2)==0)
    outputwave = 1-inputwave;
    return;
end

outputwave = 5;

== matlab function delayed_mpc_model/abc to dq0 ==
  data: ids output; iqs output; ias input; ibs input; ics input; ref_frame_position input; i0 output
function [ids,iqs,i0 ]  = fcn(ias,ibs,ics,ref_frame_position)





ids = 2/3*(ias*sin(ref_frame_position)+ibs*sin(ref_frame_position-2*pi/3)+ics*sin(ref_frame_position+2*pi/3));
iqs =  2/3*(ias*cos(ref_frame_position)+ibs*cos(ref_frame_position-2*pi/3)+ics*cos(ref_frame_position+2*pi/3));
i0 = 2/3*1/2*(ias+ibs+ics);
% iqs = (vqs-fluxlinkage_qs_derivative-ref_frame_velocity*fluxlinkage_ds)/rs;
% ids = (vds-fluxlinkage_ds_derivative+ref_frame_velocity*fluxlinkage_qs)/rs;

== matlab function delayed_mpc_model/MATLAB Function1 ==
  data: pulse input; inputwave input; outputwave output
function outputwave  = fcn(pulse, inputwave)

persistent state

if isempty(state)
state = 0;
end

if(pulse==1)
    state = state +1;
end

if(mod(state,2)==1)
    outputwave = inputwave;
    return;
end
if(mod(state,2)==0)
    outputwave = 1-inputwave;
    return;
end

outputwave = 5;
